simulink model "FIRBandpassFiltfilter"  (R2019a)
settings: Solver=VariableStepAuto  StartTime=0.0  StopTime=2*sim_time  MaxStep=1/fs  RelTol=1e-3
undefined symbols (not defined in the file): fdesignblkfcn, fs, gcbh, sim_time, tot_samples
(part 1 of 2)
settings Model: Creator=rcord  LastModifiedBy=rcord
settings DataIOCC: LoadExternalInput=on
settings DebuggingCC: UnderSpecifiedDimensionMsg=warning

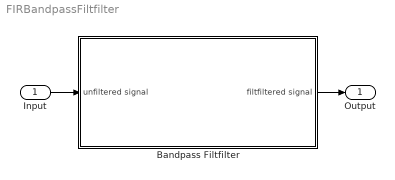
== system FIRBandpassFiltfilter ==
  Input : Inport  SampleTime=1/fs
  Bandpass Filtfilter : Subsystem  mask{fc_lo=7, fc_hi=48, trans_bw=2}
      mask prompts: fc_lo "Low Passband Frequency Corner (Hz)"; fc_hi "High Passband Frequency Corner (Hz)"; trans_bw "Transition Bandwidth (Hz)"
      mask init:
      | assignin('base','fc_lo',fc_lo)
      | assignin('base','fc_hi',fc_hi)
      | assignin('base','trans_bw',trans_bw)
      mask DialogControl DescGroupVar Prompt: Bandpass FIR Filtfilter
      mask DialogControl DescTextVar Prompt: A filtfilt bandpass operation using two identical FIR filters. The input is filtered by the first filter, reversed in time, and then filetered by the second (identical) filter. In this way there is no phase shifting and hence no group delaying. This is a non-causal operation. Both filters are created to achieve 60dB attenuation in the stopbands.
  Output : Outport
  wires:
  Bandpass Filtfilter/1(filtfiltered signal) -> Output/1
  Input/1 -> Bandpass Filtfilter/1(unfiltered signal)

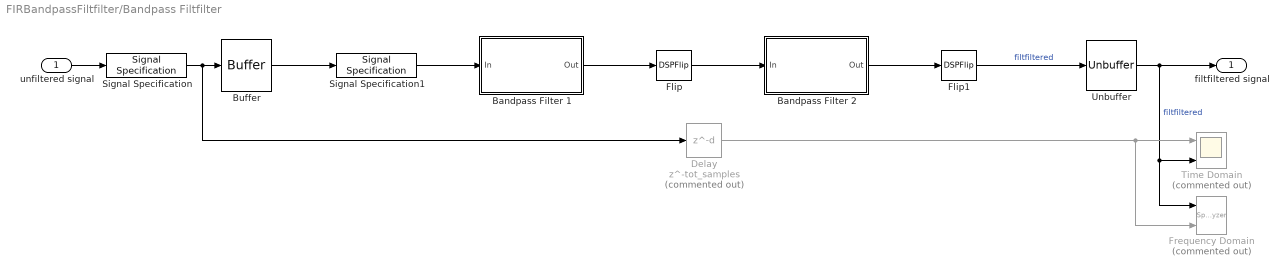
== system FIRBandpassFiltfilter/Bandpass Filtfilter ==
  unfiltered signal : Inport
  Bandpass Filter 1 : Subsystem  DialogController=fdesignblkfcn  InitFcn=fdesignblkfcn(gcbh, {'InitFcn'});  mask(Bandpass Filter){}
      mask help: Design a bandpass filter
      settings: CopyFcn=fdesignblkfcn(gcbh, {'CopyFcn'});
      mask Help: helpview(mapfilelocation('dsp'), 'dspbandpassfilter');
      mask Display: disp('Bandpass');
  Bandpass Filter 2 : Subsystem  DialogController=fdesignblkfcn  InitFcn=fdesignblkfcn(gcbh, {'InitFcn'});  mask(Bandpass Filter){}
      mask help: Design a bandpass filter
      settings: CopyFcn=fdesignblkfcn(gcbh, {'CopyFcn'});
      mask Help: helpview(mapfilelocation('dsp'), 'dspbandpassfilter');
      mask Display: disp('Bandpass');
  Buffer : Buffer  N=tot_samples  OutputFrames=off
  Delay : Delay  Commented=on  DelayLength=tot_samples
  Flip : DSPFlip
  Flip1 : DSPFlip
  Frequency Domain : SpectrumAnalyzer  Commented=on  NumInputPorts=2
  Signal Specification : SignalSpecification  Dimensions=[1 1]  SampleTime=1/fs
  Signal Specification1 : SignalSpecification  Dimensions=[tot_samples 1]  SampleTime=sim_time
  Time Domain : Scope  Commented=on  NumInputPorts=2
  Unbuffer : Unbuffer
  filtfiltered signal : Outport
  wires:
  unfiltered signal/1 -> Signal Specification/1
  Flip/1 -> Bandpass Filter 2/1(In)
  Unbuffer/1 -> filtfiltered signal/1, Frequency Domain/1, Time Domain/2  "filtfiltered"
  Buffer/1 -> Signal Specification1/1
  Flip1/1 -> Unbuffer/1  "filtfiltered"
  Bandpass Filter 1/1(Out) -> Flip/1
  Bandpass Filter 2/1(Out) -> Flip1/1
  Delay/1 -> Frequency Domain/2, Time Domain/1
  Signal Specification/1 -> Buffer/1, Delay/1
  Signal Specification1/1 -> Bandpass Filter 1/1(In)

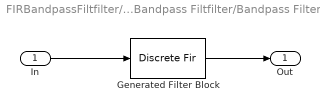
== system FIRBandpassFiltfilter/Bandpass Filtfilter/Bandpass Filter 1 ==
  In : Inport
  Generated Filter Block : DiscreteFir  Tag=BlockMethodSubSystem  Coefficients=[0.000776929510808441865 0.000512332418673175556 0.000649507731976822484 0.000783231605919231574 0.000905021318225751516 0.00100264600191827744 0.00106714069421589663 0.00108782432180463333 0.00105701691967496425 0.000965997146945759611 0.000815641873578770932 0.000602321505894979833 0.000332023194810092024 1.09800956927102187e-05 -0.000348637599893093211 -0.000733105289981374371 -0.00112487003962769504 -0.00150584800451073505 -0.00185591537398726355 -0.00215818655005050502 -0.00239466390224792611 -0.00255291159779963937 -0.00262226711623013593 -0.00259852654731812733 -0.00248109064973469707 -0.00227596105869078483 -0.00199309558074205325 -0.00164826241462783527 -0.00125897159921349415 -0.000847118183078829877 -0.000433685918532329847 -4.10844450704813259e-05 0.000311709608209888561 0.000607229989984002364 0.000833519593995551001 0.00098236117056930603 0.00105228582652108554 0.00104569468374918185 0.000971818179930198939 0.000842532437452355809 0.00067474808006303213 0.000485799697752848855 0.000295271799603360682 0.00012053980149476836 -2.18157757777684208e-05 -0.000119911371933967021 -0.000164508174703169091 -0.000152738615029307566 -8.49641961770390046e-05 3.21048344123951116e-05 0.000189340539659331626 0.000372795809019226107 0.000568018211440731889 0.000758393311444985037 0.000929415529258978391 0.00106692523455098262 0.00116138642384017664 0.00120540841667007891 0.00119756818962958762 0.00113912574433913758 0.00103715980113283971 0.000900672911691166068 0.000742839113878912506 0.000576799253401738413 0.00041759268117665696 0.000277668210174272475 0.000169078119786531791 9.91466523210604925e-05 7.32608272490951938e-05 9.10484180734499231e-05 0.00014980521715434944 0.000241569419877219599 0.000357065177342814801 0.000483373425775560691 0.000608381681675762022 0.000718576470274069753 0.000803617897789266826 0.000853816992740291636 0.000864447389584580808 0.000832721230684886366 0.000761341238602472863 0.000654932136557593138 0.000522879820984502785 0.000375130404812836946 0.000224606544635943303 8.2626552096381773e-05 -3.86733742416078916e-05 -0.000130934883241066633 -0.000186868210267593132 -0.000204302017907853216 -0.000183005264784919224 -0.000128033619509859806 -4.58871785043497458e-05 5.27502074122111666e-05 0.000157414899008992068 0.000255385581666635005 0.000336364938790588365 0.000389962669460433315 0.000410093365508195859 0.000392148844875923549 0.000336802652742026587 0.000246576585725422949 0.000128958057702035459 -7.69159971999067334e-06 -0.000151488554674454883 -0.00029160761781797434 -0.000415838855824900394 -0.000515152707347187283 -0.000581158001877931643 -0.000610261386504926335 -0.000600666224944632933 -0.000555874724427434528 -0.000481023657029473436 -0.000385787395949356972 -0.000280062544966435073 -0.000176441801146115702 -8.56445271790716185e-05 -1.88543004190929288e-05 1.66844793471682866e-05 1.50628993423606054e-05 -2.44318987436898186e-05 -0.000100517536460354275 -0.000206696441113736549 -0.000335195247654640493 -0.000474335910528225942 -0.000612956703734971776 -0.000738145475509933893 -0.000839756601368333373 -0.000908119152116288191 -0.000938205060395843715 -0.000926896848861926683 -0.000876565619263908538 -0.000791603408153504365 -0.000681310765667879977 -0.000555776612103203206 -0.000428196444672216629 -0.000310397250522012928 -0.000214917793363311857 -0.000150636329719141746 -0.000125069306253829051 -0.000140448390667110472 -0.000196660938078748772 -0.000288022367512786996 -0.00040696299144454373 -0.000541516002572591144 -0.000679594552916770907 -0.000806971598007253385 -0.000911740307014980789 -0.00098234498656469345 -0.0010118183860957186 -0.000995350786427237231 -0.000933924710617678022 -0.000831138274272268237 -0.00069605619637845605 -0.000539272845489811663 -0.000375053019317348802 -0.000216934884880757217 -7.95222247500969532e-05 2.59691509356830413e-05 8.97266964831253382e-05 0.000107380049832792859 7.73893275714320839e-05 4.3295394244580827e-06 -0.000104554949045962344 ...(+19660 chars)]  InputProcessing=Columns as channels (frame based)
  Out : Outport
  wires:
  In/1 -> Generated Filter Block/1
  Generated Filter Block/1 -> Out/1
